simulink model "Ecuacion_Diferencial_Codigo_Ejercicio_4"  (R2017b)
settings: Solver=ode1  StartTime=0.0  StopTime=10.0  RelTol=1e-3
settings Model: Creator=Elmer  LastModifiedBy=Elmer

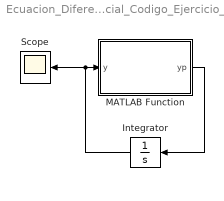
== system Ecuacion_Diferencial_Codigo_Ejercicio_4 ==
  Integrator : Integrator  InitialCondition=1
  MATLAB Function : MATLAB Function  TreatAsAtomicUnit=on
  Scope : Scope
  wires:
  MATLAB Function/1(yp) -> Integrator/1
  Integrator/1 -> Scope/1, MATLAB Function/1(y)

== matlab function Ecuacion_Diferencial_Codigo_Ejercicio_4/MATLAB Function ==
  data: y input; yp output
function yp = fcn(y)
yp= y^2 - 4;
